simulink model "SIM2"  (R2023b)
settings: Solver=ode4  StartTime=0.0  StopTime=1500  FixedStep=dt  RelTol=1e-3
InitFcn:
  | I = diag([200,200,100]);
  | Iinv = inv(I);
  | dt = 0.01;
  | dtsim = 0.1;
  | q0 = [0;0;0;1];
  | w0 = [0.05;0;0.01];
  | H0 = [0;0;0];
  | 
  | myworld = vrworld('Spacecraft.wrl');
  | open(myworld);
  | set(0,'Units','pixels');
  | scnsize = get(0,'ScreenSize');
  | f1 = vrfigure(myworld,scnsize);
StopFcn:
  | time_arr = linspace(out.tout(1), out.tout(end), size(out.w,3));
  | w_sim = reshape(out.w, size(out.w, 1), size(out.w, 3));
  | 
  | w_analytic = [.05*cos(.005*time_arr); -.05*sin(.005*time_arr); ones(1,length(time_arr))*.01];
  | 
  | plot(time_arr, w_sim - w_analytic, 'LineWidth', 2);
  | legend('\omega_1', '\omega_2', '\omega_3');
  | title('Difference Between Simulation and Analytic Results');
  | xlabel('Time (s)');
  | ylabel('Angular Velocity Difference (rad/s)');
libraries: vrlib x2, matrix_library x1
settings Model: Creator=David  LastModifiedBy=David

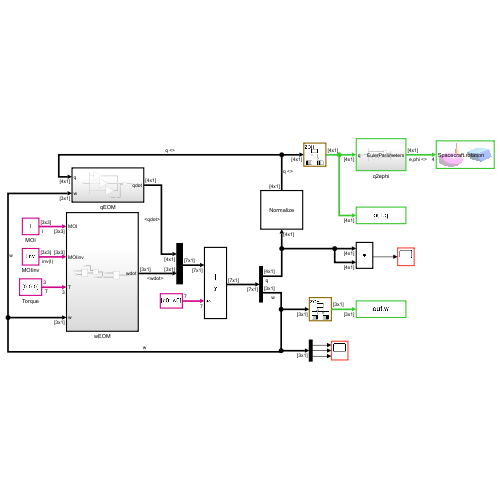
[thumbnail: Simulink's stored preview of the top-level diagram]
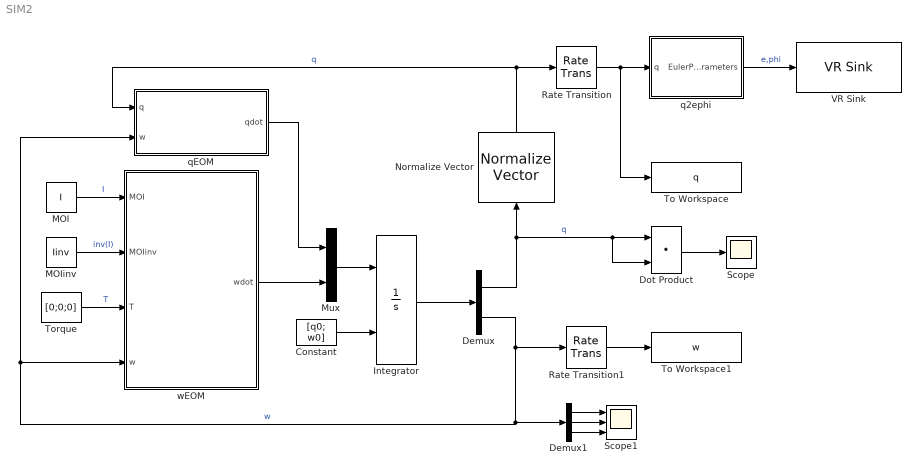
== system SIM2 ==
  Constant : Constant  Value=[q0; w0]
  Demux : Demux  Outputs=[4,3]
  Demux1 : Demux  Outputs=3
  Dot Product : DotProduct  OutDataTypeStr=Inherit: Inherit via internal rule
  Integrator : Integrator  InitialConditionSource=external
  MOI : Constant  Value=I
  MOIinv : Constant  Value=Iinv
  Mux : Mux  Inputs=2
  Normalize Vector : vrlib/Utilities/Normalize Vector  maxzero=0
  Rate Transition : RateTransition  InitialCondition=q0  OutPortSampleTime=dtsim
  Rate Transition1 : RateTransition  InitialCondition=w0  OutPortSampleTime=dtsim
  Scope : Scope
  Scope1 : Scope  NumInputPorts=3
  To Workspace : ToWorkspace  VariableName=q  SampleTime=-1
  To Workspace1 : ToWorkspace  VariableName=w  SampleTime=-1
  Torque : Constant  Value=[0;0;0]
  VR Sink : vrlib/VR Sink  InstantiateOnLoad=on  SampleTime=dtsim  ViewEnable=on  RemoteChange=off  RemoteView=off  FieldsWritten=Spacecraft.rotation.4.1.1.double  WorldFileName=Spacecraft.wrl  AutoView=off  VideoDimensions=[]  AllowVariableSize=off
  q2ephi : Subsystem
  qEOM : Subsystem
  wEOM : Subsystem
  wires:
  MOI/1 -> wEOM/1(MOI)  "I"
  MOIinv/1 -> wEOM/2(MOIinv)  "inv(I)"
  Torque/1 -> wEOM/3(T)  "T"
  Constant/1 -> Integrator/2
  Integrator/1 -> Demux/1
  Mux/1 -> Integrator/1
  q2ephi/1(EulerParameters) -> VR Sink/1  "e,phi"
  Demux/1 -> Dot Product/2, Dot Product/1, Normalize Vector/1  "q"
  wEOM/1(wdot) -> Mux/2
  Rate Transition/1 -> To Workspace/1, q2ephi/1(q)
  qEOM/1(qdot) -> Mux/1
  Demux/2 -> Demux1/1, wEOM/4(w), qEOM/2(w), Rate Transition1/1  "w"
  Normalize Vector/1 -> Rate Transition/1, qEOM/1(q)  "q"
  Rate Transition1/1 -> To Workspace1/1
  Dot Product/1 -> Scope/1
  Demux1/2 -> Scope1/2
  Demux1/1 -> Scope1/1
  Demux1/3 -> Scope1/3

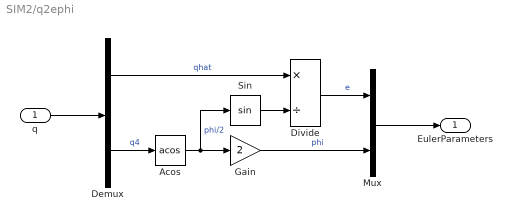
== system SIM2/q2ephi ==
  q : Inport  PortDimensions=[4;1]
  Acos : Trigonometry  Operator=acos
  Demux : Demux  Outputs=[3,1]
  Divide : Product  Inputs=*/
  Gain : Gain  Gain=2
  Mux : Mux  Inputs=2
  Sin : Trigonometry
  EulerParameters : Outport
  wires:
  q/1 -> Demux/1
  Acos/1 -> Gain/1, Sin/1  "phi/2"
  Sin/1 -> Divide/2
  Demux/1 -> Divide/1  "qhat"
  Demux/2 -> Acos/1  "q4"
  Divide/1 -> Mux/1  "e"
  Gain/1 -> Mux/2  "phi"
  Mux/1 -> EulerParameters/1

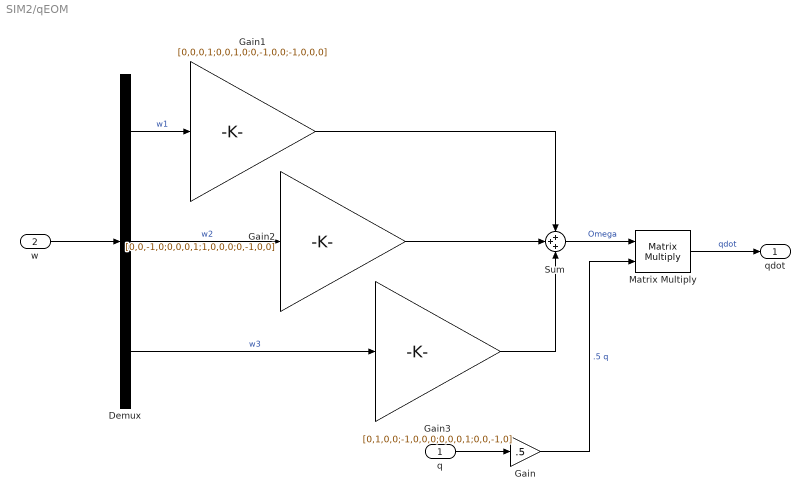
== system SIM2/qEOM ==
  q : Inport
  w : Inport  Port=2
  Demux : Demux  Outputs=3
  Gain : Gain  Gain=.5
  Gain1 : Gain  Gain=[0,0,0,1;0,0,1,0;0,-1,0,0;-1,0,0,0]
  Gain2 : Gain  Gain=[0,0,-1,0;0,0,0,1;1,0,0,0;0,-1,0,0]
  Gain3 : Gain  Gain=[0,1,0,0;-1,0,0,0;0,0,0,1;0,0,-1,0]
  Matrix Multiply : Product  Multiplication=Matrix(*)
  Sum : Sum  Inputs=+++
  qdot : Outport
  wires:
  q/1 -> Gain/1
  Matrix Multiply/1 -> qdot/1  "qdot"
  Gain/1 -> Matrix Multiply/2  ".5 q"
  w/1 -> Demux/1
  Demux/1 -> Gain1/1  "w1"
  Demux/2 -> Gain2/1  "w2"
  Demux/3 -> Gain3/1  "w3"
  Gain2/1 -> Sum/2
  Gain3/1 -> Sum/3
  Gain1/1 -> Sum/1
  Sum/1 -> Matrix Multiply/1  "Omega"

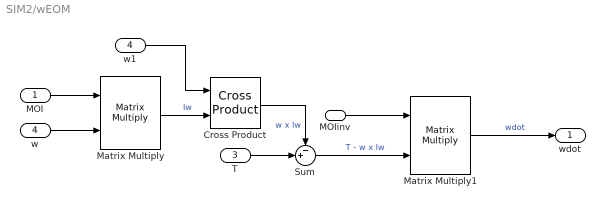
== system SIM2/wEOM ==
  MOI : Inport
  MOIinv : Inport  Port=2
  T : Inport  Port=3
  w : Inport  Port=4
  Cross Product : matrix_library/Cross Product
  Matrix Multiply : Product  Multiplication=Matrix(*)
  Matrix Multiply1 : Product  Multiplication=Matrix(*)
  Sum : Sum  Inputs=-+|
  w1 : InportShadow  Port=4
  wdot : Outport
  wires:
  T/1 -> Sum/2
  MOI/1 -> Matrix Multiply/1
  w/1 -> Matrix Multiply/2
  Matrix Multiply/1 -> Cross Product/2  "Iw"
  w1/1 -> Cross Product/1
  Cross Product/1 -> Sum/1  "w x Iw"
  MOIinv/1 -> Matrix Multiply1/1
  Sum/1 -> Matrix Multiply1/2  "T - w x Iw"
  Matrix Multiply1/1 -> wdot/1  "wdot"
